simulink model "Punto2a_simple_velocidad"  (Simulink 7.5)
settings: Solver=ode45  StartTime=0  StopTime=0.3  MaxStep=0.001  RelTol=1e-3
settings Model: Creator=Nahuek  LastModifiedBy=Nahuek

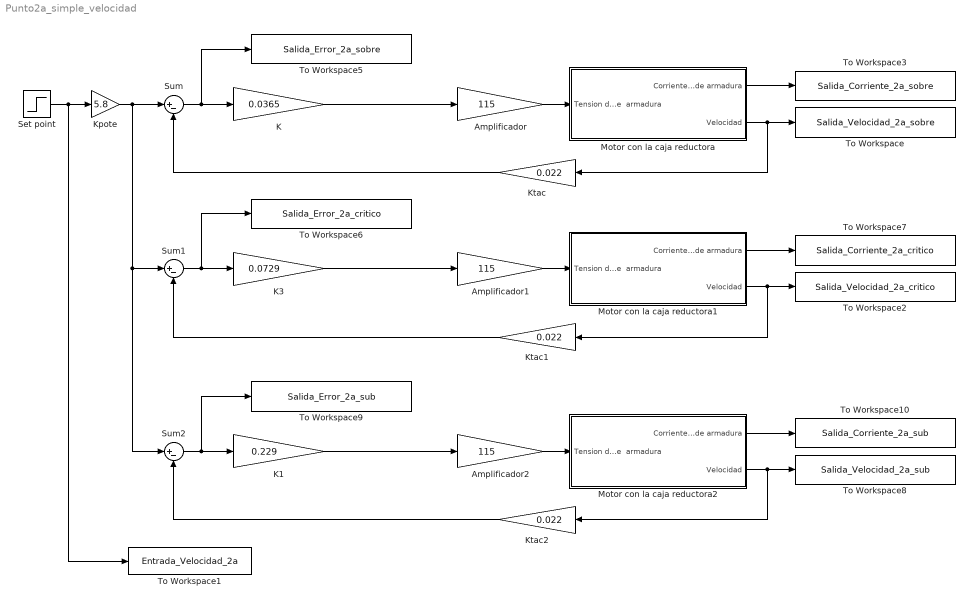
== system Punto2a_simple_velocidad ==
  Amplificador : Gain  Gain=115  ParameterDataType=fixdt(1, 16)  ParameterScaling=2^0  OutDataType=fixdt(1, 16)  OutScaling=2^0
  Amplificador1 : Gain  Gain=115  ParameterDataType=fixdt(1, 16)  ParameterScaling=2^0  OutDataType=fixdt(1, 16)  OutScaling=2^0
  Amplificador2 : Gain  Gain=115  ParameterDataType=fixdt(1, 16)  ParameterScaling=2^0  OutDataType=fixdt(1, 16)  OutScaling=2^0
  K : Gain  Gain=0.0365  ParameterDataType=fixdt(1, 16)  ParameterScaling=2^0  OutDataType=fixdt(1, 16)  OutScaling=2^0
  K1 : Gain  Gain=0.229  ParameterDataType=fixdt(1, 16)  ParameterScaling=2^0  OutDataType=fixdt(1, 16)  OutScaling=2^0
  K3 : Gain  Gain=0.0729  ParameterDataType=fixdt(1, 16)  ParameterScaling=2^0  OutDataType=fixdt(1, 16)  OutScaling=2^0
  Kpote : Gain  Gain=5.8  ParameterDataType=fixdt(1, 16)  ParameterScaling=2^0  OutDataType=fixdt(1, 16)  OutScaling=2^0
  Ktac : Gain  Gain=0.022  ParameterDataType=fixdt(1, 16)  ParameterScaling=2^0  OutDataType=fixdt(1, 16)  OutScaling=2^0
  Ktac1 : Gain  Gain=0.022  ParameterDataType=fixdt(1, 16)  ParameterScaling=2^0  OutDataType=fixdt(1, 16)  OutScaling=2^0
  Ktac2 : Gain  Gain=0.022  ParameterDataType=fixdt(1, 16)  ParameterScaling=2^0  OutDataType=fixdt(1, 16)  OutScaling=2^0
  Motor con la caja reductora : Subsystem
  Motor con la caja reductora1 : Subsystem
  Motor con la caja reductora2 : Subsystem
  Set point : Step  Time=0  SampleTime=0
  Sum : Sum  Inputs=|+-  OutDataType=fixdt(1, 16)  OutScaling=2^0
  Sum1 : Sum  Inputs=|+-  OutDataType=fixdt(1, 16)  OutScaling=2^0
  Sum2 : Sum  Inputs=|+-  OutDataType=fixdt(1, 16)  OutScaling=2^0
  To Workspace : ToWorkspace  VariableName=Salida_Velocidad_2a_sobre  SampleTime=-1  SaveFormat=Structure With Time
  To Workspace1 : ToWorkspace  VariableName=Entrada_Velocidad_2a  SampleTime=-1  SaveFormat=Structure With Time
  To Workspace10 : ToWorkspace  VariableName=Salida_Corriente_2a_sub  SampleTime=-1  SaveFormat=Structure With Time
  To Workspace2 : ToWorkspace  VariableName=Salida_Velocidad_2a_critico  SampleTime=-1  SaveFormat=Structure With Time
  To Workspace3 : ToWorkspace  VariableName=Salida_Corriente_2a_sobre  SampleTime=-1  SaveFormat=Structure With Time
  To Workspace5 : ToWorkspace  VariableName=Salida_Error_2a_sobre  SampleTime=-1  SaveFormat=Structure With Time
  To Workspace6 : ToWorkspace  VariableName=Salida_Error_2a_critico  SampleTime=-1  SaveFormat=Structure With Time
  To Workspace7 : ToWorkspace  VariableName=Salida_Corriente_2a_critico  SampleTime=-1  SaveFormat=Structure With Time
  To Workspace8 : ToWorkspace  VariableName=Salida_Velocidad_2a_sub  SampleTime=-1  SaveFormat=Structure With Time
  To Workspace9 : ToWorkspace  VariableName=Salida_Error_2a_sub  SampleTime=-1  SaveFormat=Structure With Time
  wires:
  Sum/1 -> K/1, To Workspace5/1
  Amplificador/1 -> Motor con la caja reductora/1(Tension de  armadura)
  Motor con la caja reductora/2(Velocidad) -> To Workspace/1, Ktac/1
  Ktac/1 -> Sum/2
  Kpote/1 -> Sum/1, Sum1/1, Sum2/1
  Set point/1 -> Kpote/1, To Workspace1/1
  K/1 -> Amplificador/1
  Motor con la caja reductora/1(Corriente de armadura) -> To Workspace3/1
  Sum1/1 -> K3/1, To Workspace6/1
  Amplificador1/1 -> Motor con la caja reductora1/1(Tension de  armadura)
  Motor con la caja reductora1/2(Velocidad) -> Ktac1/1, To Workspace2/1
  Ktac1/1 -> Sum1/2
  K3/1 -> Amplificador1/1
  Motor con la caja reductora1/1(Corriente de armadura) -> To Workspace7/1
  Sum2/1 -> K1/1, To Workspace9/1
  Amplificador2/1 -> Motor con la caja reductora2/1(Tension de  armadura)
  Motor con la caja reductora2/2(Velocidad) -> Ktac2/1, To Workspace8/1
  Ktac2/1 -> Sum2/2
  K1/1 -> Amplificador2/1
  Motor con la caja reductora2/1(Corriente de armadura) -> To Workspace10/1

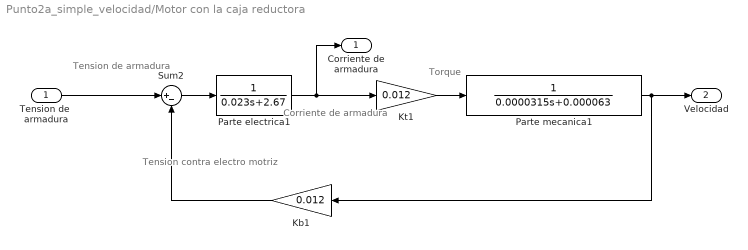
== system Punto2a_simple_velocidad/Motor con la caja reductora ==
  note: Tension contra
      |  electro motriz
  note: Corriente de
      | armadura
  note: Torque
  note: Tension de
      |  armadura
  Tension de  armadura : Inport
  Kb1 : Gain  Gain=0.012  ParameterDataType=fixdt(1, 16)  ParameterScaling=2^0  OutDataType=fixdt(1, 16)  OutScaling=2^0
  Kt1 : Gain  Gain=0.012  ParameterDataType=fixdt(1, 16)  ParameterScaling=2^0  OutDataType=fixdt(1, 16)  OutScaling=2^0
  Parte electrica1 : TransferFcn  Denominator=[0.023 2.67]
  Parte mecanica1 : TransferFcn  Denominator=[0.0000315 0.000063]
  Sum2 : Sum  Inputs=|+-  OutDataType=fixdt(1, 16)  OutScaling=2^0
  Corriente de armadura : Outport
  Velocidad : Outport  Port=2
  wires:
  Sum2/1 -> Parte electrica1/1
  Kt1/1 -> Parte mecanica1/1
  Parte electrica1/1 -> Kt1/1, Corriente de armadura/1
  Kb1/1 -> Sum2/2
  Parte mecanica1/1 -> Kb1/1, Velocidad/1
  Tension de  armadura/1 -> Sum2/1

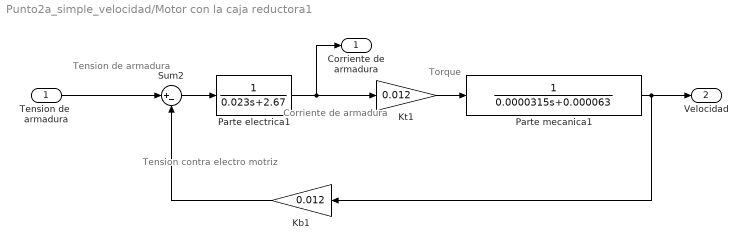
== system Punto2a_simple_velocidad/Motor con la caja reductora1 ==
  note: Tension contra
      |  electro motriz
  note: Corriente de
      | armadura
  note: Torque
  note: Tension de
      |  armadura
  Tension de  armadura : Inport
  Kb1 : Gain  Gain=0.012  ParameterDataType=fixdt(1, 16)  ParameterScaling=2^0  OutDataType=fixdt(1, 16)  OutScaling=2^0
  Kt1 : Gain  Gain=0.012  ParameterDataType=fixdt(1, 16)  ParameterScaling=2^0  OutDataType=fixdt(1, 16)  OutScaling=2^0
  Parte electrica1 : TransferFcn  Denominator=[0.023 2.67]
  Parte mecanica1 : TransferFcn  Denominator=[0.0000315 0.000063]
  Sum2 : Sum  Inputs=|+-  OutDataType=fixdt(1, 16)  OutScaling=2^0
  Corriente de armadura : Outport
  Velocidad : Outport  Port=2
  wires:
  Sum2/1 -> Parte electrica1/1
  Kt1/1 -> Parte mecanica1/1
  Parte electrica1/1 -> Kt1/1, Corriente de armadura/1
  Kb1/1 -> Sum2/2
  Parte mecanica1/1 -> Kb1/1, Velocidad/1
  Tension de  armadura/1 -> Sum2/1

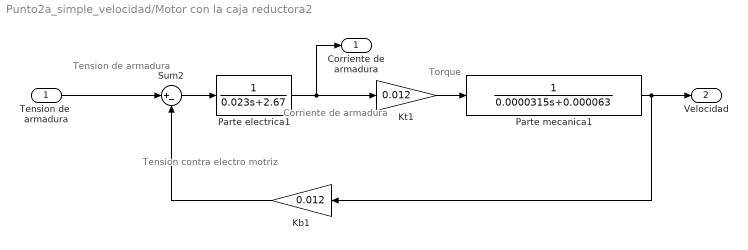
== system Punto2a_simple_velocidad/Motor con la caja reductora2 ==
  note: Tension contra
      |  electro motriz
  note: Corriente de
      | armadura
  note: Torque
  note: Tension de
      |  armadura
  Tension de  armadura : Inport
  Kb1 : Gain  Gain=0.012  ParameterDataType=fixdt(1, 16)  ParameterScaling=2^0  OutDataType=fixdt(1, 16)  OutScaling=2^0
  Kt1 : Gain  Gain=0.012  ParameterDataType=fixdt(1, 16)  ParameterScaling=2^0  OutDataType=fixdt(1, 16)  OutScaling=2^0
  Parte electrica1 : TransferFcn  Denominator=[0.023 2.67]
  Parte mecanica1 : TransferFcn  Denominator=[0.0000315 0.000063]
  Sum2 : Sum  Inputs=|+-  OutDataType=fixdt(1, 16)  OutScaling=2^0
  Corriente de armadura : Outport
  Velocidad : Outport  Port=2
  wires:
  Sum2/1 -> Parte electrica1/1
  Kt1/1 -> Parte mecanica1/1
  Parte electrica1/1 -> Kt1/1, Corriente de armadura/1
  Kb1/1 -> Sum2/2
  Parte mecanica1/1 -> Kb1/1, Velocidad/1
  Tension de  armadura/1 -> Sum2/1
